simulink model "omav_eom"  (R2020a)
settings: Solver=VariableStepAuto  StartTime=0.0  StopTime=10.0  RelTol=1e-3
undefined symbols (not defined in the file): params
libraries: vrlib x2
settings Model: Creator=daniel  LastModifiedBy=daniel

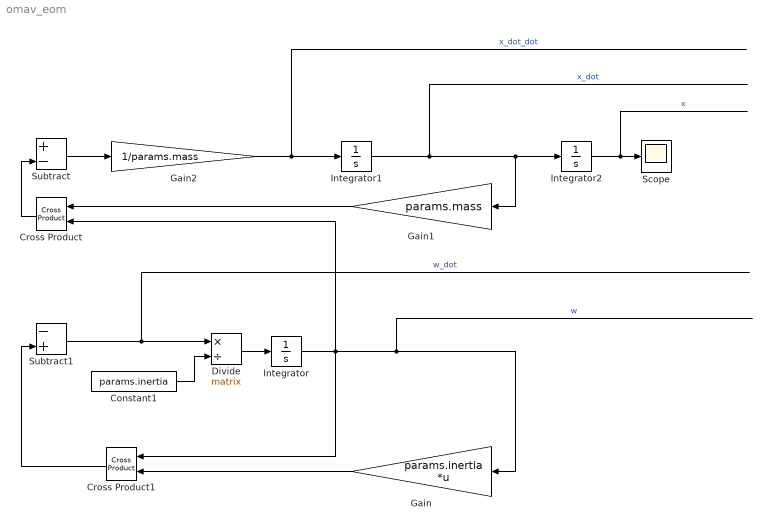
== system omav_eom ==
  Constant1 : Constant  Value=params.inertia  VectorParams1D=off
  Cross Product : vrlib/Utilities/Cross Product
  Cross Product1 : vrlib/Utilities/Cross Product
  Divide : Product  Inputs=*/  Multiplication=Matrix(*)
  Gain : Gain  Gain=params.inertia  Multiplication=Matrix(K*u) (u vector)
  Gain1 : Gain  Gain=params.mass
  Gain2 : Gain  Gain=1/params.mass
  Integrator : Integrator
  Integrator1 : Integrator
  Integrator2 : Integrator
  Scope : Scope
  Subtract : Sum  Inputs=+-
  Subtract1 : Sum  Inputs=-+
  wires:
  Integrator1/1 -> Gain1/1, Integrator2/1  "x_dot"
  Integrator2/1 -> Scope/1  "x"
  Gain2/1 -> Integrator1/1  "x_dot_dot"
  Integrator/1 -> Gain/1, Cross Product1/1, Cross Product/2  "w"
  Subtract1/1 -> Divide/1  "w_dot"
  Gain1/1 -> Cross Product/1
  Subtract/1 -> Gain2/1
  Gain/1 -> Cross Product1/2
  Cross Product1/1 -> Subtract1/2
  Cross Product/1 -> Subtract/2
  Divide/1 -> Integrator/1
  Constant1/1 -> Divide/2
  ? -> Subtract1/1  "torque_b"
  ? -> Subtract/1  "force_b"
